simulink model "SIMControlleurMAT"  (Simulink 8.8)
settings: Solver=ode45  StartTime=0.0  StopTime=50  RelTol=1e-3  EnableMultiTasking=on
libraries: simulink x2
settings Model: Creator=Utilisateur-pc  LastModifiedBy=Jérôme
settings OptimizationCC: ExpressionDepthLimit=2147483647
settings DebuggingCC: SolverPrmCheckMsg=warning

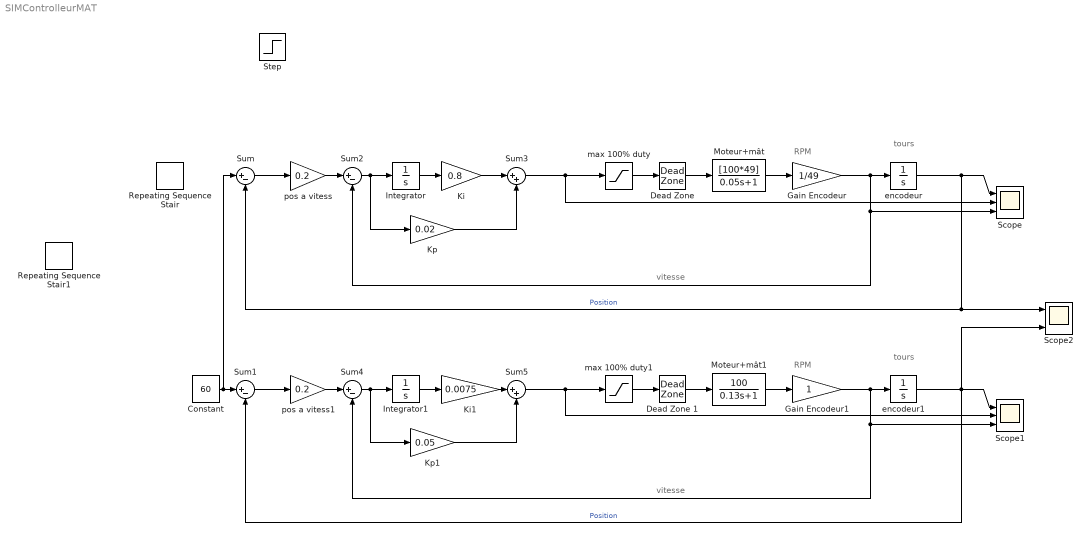
== system SIMControlleurMAT ==
  note: RPM
  note: tours
  note: vitesse
  note: RPM
  note: tours
  note: vitesse
  Constant : Constant  Value=60  SampleTime=0.1
  "Dead Zone " : DeadZone  LowerValue=-0.1  UpperValue=0.1  SaturateOnIntegerOverflow=on
  Dead Zone 1 : DeadZone  LowerValue=-0.1  UpperValue=0.1  SaturateOnIntegerOverflow=on
  Gain Encodeur : Gain  Gain=1/49
  Gain Encodeur1 : Gain
  Integrator : Integrator
  Integrator1 : Integrator
  Ki : Gain  Gain=0.8
  Ki1 : Gain  Gain=0.0075
  Kp : Gain  Gain=0.02
  Kp1 : Gain  Gain=0.05
  Moteur+mât : TransferFcn  Numerator=[100*49]  Denominator=[0.05 1]
  Moteur+mât1 : TransferFcn  Numerator=[100]  Denominator=[0.13 1]
  Repeating Sequence Stair : simulink/Sources/Repeating Sequence Stair  OutValues=[-170 170].'  tsamp=50  OutMin=[]  OutMax=[]  OutDataTypeStr=double  OutputDataTypeScalingMode=double  OutDataType=fixdt(0,8)  ConRadixGroup=Best Precision: Vector-wise  OutScaling=2^-12
  Repeating Sequence Stair1 : simulink/Sources/Repeating Sequence Stair  OutValues=[-170 170].'  tsamp=50  OutMin=[]  OutMax=[]  OutDataTypeStr=double  OutputDataTypeScalingMode=double  OutDataType=fixdt(0,8)  ConRadixGroup=Best Precision: Vector-wise  OutScaling=2^-12
  Scope : Scope  NumInputPorts=3
  Scope1 : Scope  NumInputPorts=3
  Scope2 : Scope  NumInputPorts=2
  Step : Step  Time=120  Before=-170  After=170  SampleTime=0.1  ZeroCross=off
  Sum : Sum  Inputs=|+-  SampleTime=0.1
  Sum1 : Sum  Inputs=|+-  SampleTime=0.1
  Sum2 : Sum  Inputs=|+-
  Sum3 : Sum  Inputs=|++
  Sum4 : Sum  Inputs=|+-
  Sum5 : Sum  Inputs=|++
  encodeur : Integrator
  encodeur1 : Integrator
  max 100% duty : Saturate  UpperLimit=1  LowerLimit=-1
  max 100% duty1 : Saturate  UpperLimit=1  LowerLimit=-1
  pos a vitess : Gain  Gain=0.2
  pos a vitess1 : Gain  Gain=0.2
  wires:
  Moteur+mât/1 -> Gain Encodeur/1
  encodeur/1 -> Scope/1, Scope2/1, Sum/2  "Position"
  max 100% duty/1 -> "Dead Zone "/1
  "Dead Zone "/1 -> Moteur+mât/1
  pos a vitess/1 -> Sum2/1
  Sum2/1 -> Integrator/1, Kp/1
  Gain Encodeur/1 -> Scope/3, Sum2/2, encodeur/1
  Integrator/1 -> Ki/1
  Sum3/1 -> max 100% duty/1, Scope/2
  Kp/1 -> Sum3/2
  Sum/1 -> pos a vitess/1
  Ki/1 -> Sum3/1
  Moteur+mât1/1 -> Gain Encodeur1/1
  encodeur1/1 -> Scope2/2, Scope1/1, Sum1/2  "Position"
  max 100% duty1/1 -> Dead Zone 1/1
  Dead Zone 1/1 -> Moteur+mât1/1
  pos a vitess1/1 -> Sum4/1
  Sum4/1 -> Integrator1/1, Kp1/1
  Gain Encodeur1/1 -> Scope1/3, Sum4/2, encodeur1/1
  Integrator1/1 -> Ki1/1
  Sum5/1 -> max 100% duty1/1, Scope1/2
  Kp1/1 -> Sum5/2
  Sum1/1 -> pos a vitess1/1
  Ki1/1 -> Sum5/1
  Constant/1 -> Sum/1, Sum1/1
